simulink model "cruise_control"  (R2020b)
settings: Solver=VariableStepAuto  StartTime=0.0  StopTime=10.0  RelTol=1e-3
undefined symbols (not defined in the file or in its folder): B, M
settings Model: DataDictionary=cruise_model_cum_controller_parametrs.sldd  Creator=153  LastModifiedBy=153

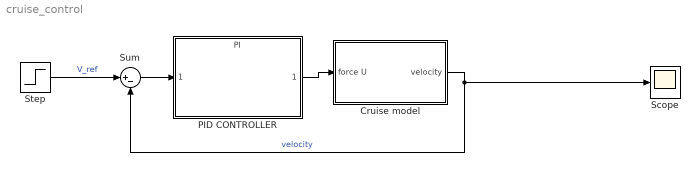
== system cruise_control ==
  Cruise model : Subsystem
  PID CONTROLLER : ModelReference  ModelNameDialog=PI  SimulationMode=Normal  ModelReferenceVersion=1.5
  Scope : Scope
  Step : Step  Time=0  After=10  SampleTime=0
  Sum : Sum  Inputs=|+-
  wires:
  Cruise model/1(velocity) -> Sum/2, Scope/1  "velocity"
  Step/1 -> Sum/1  "V_ref"
  Sum/1 -> PID CONTROLLER/1
  PID CONTROLLER/1 -> Cruise model/1(force U)

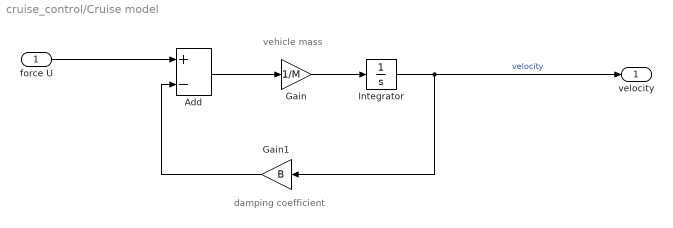
== system cruise_control/Cruise model ==
  note: vehicle mass
  note: damping coefficient
  force U : Inport
  Add : Sum  Inputs=+-
  Gain : Gain  Gain=1/M
  Gain1 : Gain  Gain=B
  Integrator : Integrator
  velocity : Outport
  wires:
  Gain/1 -> Integrator/1
  Add/1 -> Gain/1
  force U/1 -> Add/1
  Integrator/1 -> velocity/1, Gain1/1  "velocity"
  Gain1/1 -> Add/2
